simulink model "Robot"  (R2022b)
settings: Solver=FixedStepDiscrete  StartTime=0.0  StopTime=30  FixedStep=0.001  RelTol=1e-3
InitFcn:
  | load("BusConfig.mat");
undefined symbols (not defined in the file or in its folder): DiscIntNeverNeededParam
libraries: slrealtimeethercatlib x119, simulink x20
(part 6 of 7)

== system Robot/Motor3 Torque Control Init Frame/SDO Set 0x6098:35 Frame/If Action Subsystem6 ==
  In1 : Inport
  Action Port : ActionPort
  Out1 : Outport
  wires:
  In1/1 -> Out1/1

== system Robot/Motor3 Torque Control Init Frame/SDO Set 0x6098:35 Frame/If Action Subsystem7 ==
  In1 : Inport
  Action Port : ActionPort
  Discrete-Time Integrator : DiscreteIntegrator  SampleTime=-1  ICPrevOutput=DiscIntNeverNeededParam  ICPrevScaledInput=DiscIntNeverNeededParam
  Out1 : Outport
  wires:
  In1/1 -> Discrete-Time Integrator/1
  Discrete-Time Integrator/1 -> Out1/1

== system Robot/Motor3 Torque Control Init Frame/Set MasterState to OP Frame/If Action Subsystem5 ==
  In1 : Inport
  Action Port : ActionPort  ActionPortLabel=if((u1 > 0.1))
  Out1 : Outport
  wires:
  In1/1 -> Out1/1

== system Robot/Motor3 Torque Control Init Frame/Set MasterState to OP Frame/If Action Subsystem6 ==
  In1 : Inport
  Action Port : ActionPort  ActionPortLabel=else
  Out1 : Outport
  wires:
  In1/1 -> Out1/1

== system Robot/Motor3 Torque Control Init Frame/Set MasterState to OP Frame/If Action Subsystem7 ==
  In1 : Inport
  Action Port : ActionPort  ActionPortLabel=if((u1 == 8))
  Discrete-Time Integrator : DiscreteIntegrator  SampleTime=-1  ICPrevOutput=DiscIntNeverNeededParam  ICPrevScaledInput=DiscIntNeverNeededParam
  Out1 : Outport
  wires:
  In1/1 -> Discrete-Time Integrator/1
  Discrete-Time Integrator/1 -> Out1/1

== system Robot/Motor3 Torque Control Init Frame/Set MasterState to SafeOP Frame/If Action Subsystem5 ==
  In1 : Inport
  Action Port : ActionPort  ActionPortLabel=if((u1 > 0.1))
  Out1 : Outport
  wires:
  In1/1 -> Out1/1

== system Robot/Motor3 Torque Control Init Frame/Set MasterState to SafeOP Frame/If Action Subsystem6 ==
  In1 : Inport
  Action Port : ActionPort  ActionPortLabel=else
  Out1 : Outport
  wires:
  In1/1 -> Out1/1

== system Robot/Motor3 Torque Control Init Frame/Set MasterState to SafeOP Frame/If Action Subsystem7 ==
  In1 : Inport
  Action Port : ActionPort  ActionPortLabel=if((u1 == 4))
  Discrete-Time Integrator : DiscreteIntegrator  SampleTime=-1  ICPrevOutput=DiscIntNeverNeededParam  ICPrevScaledInput=DiscIntNeverNeededParam
  Out1 : Outport
  wires:
  In1/1 -> Discrete-Time Integrator/1
  Discrete-Time Integrator/1 -> Out1/1

== system Robot/Motor3 Torque Control Init Frame/State_10_Enable/Subsystem ==
  Case : Inport
  Case Default : Inport  Port=2
  Constant : Constant
  Constant1 : Constant  Value=0
  Constant2 : Constant  Value=TaskIndex
  Merge : Merge
  Switch Case Action Subsystem : Subsystem  TreatAsAtomicUnit=on
  Switch Case Action Subsystem1 : Subsystem  TreatAsAtomicUnit=on
  Enable : Outport
  FinishIndex : Outport  Port=2
  wires:
  Constant/1 -> Switch Case Action Subsystem/1(In1)
  Case/1 -> Switch Case Action Subsystem/Action
  Switch Case Action Subsystem/1(Out1) -> Merge/1
  Merge/1 -> Enable/1
  Case Default/1 -> Switch Case Action Subsystem1/Action
  Constant1/1 -> Switch Case Action Subsystem1/1(In1)
  Switch Case Action Subsystem1/1(Default) -> Merge/2
  Constant2/1 -> FinishIndex/1

== system Robot/Motor3 Torque Control Init Frame/State_11_Enable/Subsystem ==
  Case : Inport
  Case Default : Inport  Port=2
  Constant : Constant
  Constant1 : Constant  Value=0
  Constant2 : Constant  Value=TaskIndex
  Merge : Merge
  Switch Case Action Subsystem : Subsystem  TreatAsAtomicUnit=on
  Switch Case Action Subsystem1 : Subsystem  TreatAsAtomicUnit=on
  Enable : Outport
  FinishIndex : Outport  Port=2
  wires:
  Constant/1 -> Switch Case Action Subsystem/1(In1)
  Case/1 -> Switch Case Action Subsystem/Action
  Switch Case Action Subsystem/1(Out1) -> Merge/1
  Merge/1 -> Enable/1
  Case Default/1 -> Switch Case Action Subsystem1/Action
  Constant1/1 -> Switch Case Action Subsystem1/1(In1)
  Switch Case Action Subsystem1/1(Default) -> Merge/2
  Constant2/1 -> FinishIndex/1

== system Robot/Motor3 Torque Control Init Frame/State_12_Enable/Subsystem ==
  Case : Inport
  Case Default : Inport  Port=2
  Constant : Constant
  Constant1 : Constant  Value=0
  Constant2 : Constant  Value=TaskIndex
  Merge : Merge
  Switch Case Action Subsystem : Subsystem  TreatAsAtomicUnit=on
  Switch Case Action Subsystem1 : Subsystem  TreatAsAtomicUnit=on
  Enable : Outport
  FinishIndex : Outport  Port=2
  wires:
  Constant/1 -> Switch Case Action Subsystem/1(In1)
  Case/1 -> Switch Case Action Subsystem/Action
  Switch Case Action Subsystem/1(Out1) -> Merge/1
  Merge/1 -> Enable/1
  Case Default/1 -> Switch Case Action Subsystem1/Action
  Constant1/1 -> Switch Case Action Subsystem1/1(In1)
  Switch Case Action Subsystem1/1(Default) -> Merge/2
  Constant2/1 -> FinishIndex/1

== system Robot/Motor3 Torque Control Init Frame/State_13_Enable/Subsystem ==
  Case : Inport
  Case Default : Inport  Port=2
  Constant : Constant
  Constant1 : Constant  Value=0
  Constant2 : Constant  Value=TaskIndex
  Merge : Merge
  Switch Case Action Subsystem : Subsystem  TreatAsAtomicUnit=on
  Switch Case Action Subsystem1 : Subsystem  TreatAsAtomicUnit=on
  Enable : Outport
  FinishIndex : Outport  Port=2
  wires:
  Constant/1 -> Switch Case Action Subsystem/1(In1)
  Case/1 -> Switch Case Action Subsystem/Action
  Switch Case Action Subsystem/1(Out1) -> Merge/1
  Merge/1 -> Enable/1
  Case Default/1 -> Switch Case Action Subsystem1/Action
  Constant1/1 -> Switch Case Action Subsystem1/1(In1)
  Switch Case Action Subsystem1/1(Default) -> Merge/2
  Constant2/1 -> FinishIndex/1

== system Robot/Motor3 Torque Control Init Frame/State_1_Enable/Subsystem ==
  Case : Inport
  Case Default : Inport  Port=2
  Constant : Constant
  Constant1 : Constant  Value=0
  Constant2 : Constant  Value=TaskIndex
  Merge : Merge
  Switch Case Action Subsystem : Subsystem  TreatAsAtomicUnit=on
  Switch Case Action Subsystem1 : Subsystem  TreatAsAtomicUnit=on
  Enable : Outport
  FinishIndex : Outport  Port=2
  wires:
  Constant/1 -> Switch Case Action Subsystem/1(In1)
  Case/1 -> Switch Case Action Subsystem/Action
  Switch Case Action Subsystem/1(Out1) -> Merge/1
  Merge/1 -> Enable/1
  Case Default/1 -> Switch Case Action Subsystem1/Action
  Constant1/1 -> Switch Case Action Subsystem1/1(In1)
  Switch Case Action Subsystem1/1(Default) -> Merge/2
  Constant2/1 -> FinishIndex/1

== system Robot/Motor3 Torque Control Init Frame/State_2_Enable/Subsystem ==
  Case : Inport
  Case Default : Inport  Port=2
  Constant : Constant
  Constant1 : Constant  Value=0
  Constant2 : Constant  Value=TaskIndex
  Merge : Merge
  Switch Case Action Subsystem : Subsystem  TreatAsAtomicUnit=on
  Switch Case Action Subsystem1 : Subsystem  TreatAsAtomicUnit=on
  Enable : Outport
  FinishIndex : Outport  Port=2
  wires:
  Constant/1 -> Switch Case Action Subsystem/1(In1)
  Case/1 -> Switch Case Action Subsystem/Action
  Switch Case Action Subsystem/1(Out1) -> Merge/1
  Merge/1 -> Enable/1
  Case Default/1 -> Switch Case Action Subsystem1/Action
  Constant1/1 -> Switch Case Action Subsystem1/1(In1)
  Switch Case Action Subsystem1/1(Default) -> Merge/2
  Constant2/1 -> FinishIndex/1

== system Robot/Motor3 Torque Control Init Frame/State_3_Enable/Subsystem ==
  Case : Inport
  Case Default : Inport  Port=2
  Constant : Constant
  Constant1 : Constant  Value=0
  Constant2 : Constant  Value=TaskIndex
  Merge : Merge
  Switch Case Action Subsystem : Subsystem  TreatAsAtomicUnit=on
  Switch Case Action Subsystem1 : Subsystem  TreatAsAtomicUnit=on
  Enable : Outport
  FinishIndex : Outport  Port=2
  wires:
  Constant/1 -> Switch Case Action Subsystem/1(In1)
  Case/1 -> Switch Case Action Subsystem/Action
  Switch Case Action Subsystem/1(Out1) -> Merge/1
  Merge/1 -> Enable/1
  Case Default/1 -> Switch Case Action Subsystem1/Action
  Constant1/1 -> Switch Case Action Subsystem1/1(In1)
  Switch Case Action Subsystem1/1(Default) -> Merge/2
  Constant2/1 -> FinishIndex/1

== system Robot/Motor3 Torque Control Init Frame/State_4_Enable/Subsystem ==
  Case : Inport
  Case Default : Inport  Port=2
  Constant : Constant
  Constant1 : Constant  Value=0
  Constant2 : Constant  Value=TaskIndex
  Merge : Merge
  Switch Case Action Subsystem : Subsystem  TreatAsAtomicUnit=on
  Switch Case Action Subsystem1 : Subsystem  TreatAsAtomicUnit=on
  Enable : Outport
  FinishIndex : Outport  Port=2
  wires:
  Constant/1 -> Switch Case Action Subsystem/1(In1)
  Case/1 -> Switch Case Action Subsystem/Action
  Switch Case Action Subsystem/1(Out1) -> Merge/1
  Merge/1 -> Enable/1
  Case Default/1 -> Switch Case Action Subsystem1/Action
  Constant1/1 -> Switch Case Action Subsystem1/1(In1)
  Switch Case Action Subsystem1/1(Default) -> Merge/2
  Constant2/1 -> FinishIndex/1

== system Robot/Motor3 Torque Control Init Frame/State_5_Enable/Subsystem ==
  Case : Inport
  Case Default : Inport  Port=2
  Constant : Constant
  Constant1 : Constant  Value=0
  Constant2 : Constant  Value=TaskIndex
  Merge : Merge
  Switch Case Action Subsystem : Subsystem  TreatAsAtomicUnit=on
  Switch Case Action Subsystem1 : Subsystem  TreatAsAtomicUnit=on
  Enable : Outport
  FinishIndex : Outport  Port=2
  wires:
  Constant/1 -> Switch Case Action Subsystem/1(In1)
  Case/1 -> Switch Case Action Subsystem/Action
  Switch Case Action Subsystem/1(Out1) -> Merge/1
  Merge/1 -> Enable/1
  Case Default/1 -> Switch Case Action Subsystem1/Action
  Constant1/1 -> Switch Case Action Subsystem1/1(In1)
  Switch Case Action Subsystem1/1(Default) -> Merge/2
  Constant2/1 -> FinishIndex/1

== system Robot/Motor3 Torque Control Init Frame/State_6_Enable/Subsystem ==
  Case : Inport
  Case Default : Inport  Port=2
  Constant : Constant
  Constant1 : Constant  Value=0
  Constant2 : Constant  Value=TaskIndex
  Merge : Merge
  Switch Case Action Subsystem : Subsystem  TreatAsAtomicUnit=on
  Switch Case Action Subsystem1 : Subsystem  TreatAsAtomicUnit=on
  Enable : Outport
  FinishIndex : Outport  Port=2
  wires:
  Constant/1 -> Switch Case Action Subsystem/1(In1)
  Case/1 -> Switch Case Action Subsystem/Action
  Switch Case Action Subsystem/1(Out1) -> Merge/1
  Merge/1 -> Enable/1
  Case Default/1 -> Switch Case Action Subsystem1/Action
  Constant1/1 -> Switch Case Action Subsystem1/1(In1)
  Switch Case Action Subsystem1/1(Default) -> Merge/2
  Constant2/1 -> FinishIndex/1

== system Robot/Motor3 Torque Control Init Frame/State_7_Enable/Subsystem ==
  Case : Inport
  Case Default : Inport  Port=2
  Constant : Constant
  Constant1 : Constant  Value=0
  Constant2 : Constant  Value=TaskIndex
  Merge : Merge
  Switch Case Action Subsystem : Subsystem  TreatAsAtomicUnit=on
  Switch Case Action Subsystem1 : Subsystem  TreatAsAtomicUnit=on
  Enable : Outport
  FinishIndex : Outport  Port=2
  wires:
  Constant/1 -> Switch Case Action Subsystem/1(In1)
  Case/1 -> Switch Case Action Subsystem/Action
  Switch Case Action Subsystem/1(Out1) -> Merge/1
  Merge/1 -> Enable/1
  Case Default/1 -> Switch Case Action Subsystem1/Action
  Constant1/1 -> Switch Case Action Subsystem1/1(In1)
  Switch Case Action Subsystem1/1(Default) -> Merge/2
  Constant2/1 -> FinishIndex/1

== system Robot/Motor3 Torque Control Init Frame/State_8_Enable/Subsystem ==
  Case : Inport
  Case Default : Inport  Port=2
  Constant : Constant
  Constant1 : Constant  Value=0
  Constant2 : Constant  Value=TaskIndex
  Merge : Merge
  Switch Case Action Subsystem : Subsystem  TreatAsAtomicUnit=on
  Switch Case Action Subsystem1 : Subsystem  TreatAsAtomicUnit=on
  Enable : Outport
  FinishIndex : Outport  Port=2
  wires:
  Constant/1 -> Switch Case Action Subsystem/1(In1)
  Case/1 -> Switch Case Action Subsystem/Action
  Switch Case Action Subsystem/1(Out1) -> Merge/1
  Merge/1 -> Enable/1
  Case Default/1 -> Switch Case Action Subsystem1/Action
  Constant1/1 -> Switch Case Action Subsystem1/1(In1)
  Switch Case Action Subsystem1/1(Default) -> Merge/2
  Constant2/1 -> FinishIndex/1

== system Robot/Motor3 Torque Control Init Frame/State_9_Enable/Subsystem ==
  Case : Inport
  Case Default : Inport  Port=2
  Constant : Constant
  Constant1 : Constant  Value=0
  Constant2 : Constant  Value=TaskIndex
  Merge : Merge
  Switch Case Action Subsystem : Subsystem  TreatAsAtomicUnit=on
  Switch Case Action Subsystem1 : Subsystem  TreatAsAtomicUnit=on
  Enable : Outport
  FinishIndex : Outport  Port=2
  wires:
  Constant/1 -> Switch Case Action Subsystem/1(In1)
  Case/1 -> Switch Case Action Subsystem/Action
  Switch Case Action Subsystem/1(Out1) -> Merge/1
  Merge/1 -> Enable/1
  Case Default/1 -> Switch Case Action Subsystem1/Action
  Constant1/1 -> Switch Case Action Subsystem1/1(In1)
  Switch Case Action Subsystem1/1(Default) -> Merge/2
  Constant2/1 -> FinishIndex/1

== system Robot/Motor4 Torque Control Init Frame/Get MasterState OP Frame/If Action Subsystem5 ==
  In1 : Inport
  Action Port : ActionPort  ActionPortLabel=if((u1 == 8))
  Out1 : Outport
  wires:
  In1/1 -> Out1/1

== system Robot/Motor4 Torque Control Init Frame/Get MasterState OP Frame/If Action Subsystem6 ==
  In1 : Inport
  Action Port : ActionPort  ActionPortLabel=else
  Out1 : Outport
  wires:
  In1/1 -> Out1/1

== system Robot/Motor4 Torque Control Init Frame/Get MasterState OP Frame/If Action Subsystem7 ==
  In1 : Inport
  Action Port : ActionPort  ActionPortLabel=if((u1 == 4663))
  Discrete-Time Integrator : DiscreteIntegrator  SampleTime=-1  ICPrevOutput=DiscIntNeverNeededParam  ICPrevScaledInput=DiscIntNeverNeededParam
  Out1 : Outport
  wires:
  In1/1 -> Discrete-Time Integrator/1
  Discrete-Time Integrator/1 -> Out1/1

== system Robot/Motor4 Torque Control Init Frame/PDO Set 0x6040:6->7->15 Frame/If Action Subsystem ==
  In1 : Inport
  Action Port : ActionPort  ActionPortLabel=if((u1 == 720)&(u2 == 500))
  Out1 : Outport
  wires:
  In1/1 -> Out1/1

== system Robot/Motor4 Torque Control Init Frame/PDO Set 0x6040:6->7->15 Frame/If Action Subsystem1 ==
  In1 : Inport
  Action Port : ActionPort  ActionPortLabel=elseif((u1 == 689)&(u2 == 500))
  Out1 : Outport
  wires:
  In1/1 -> Out1/1

== system Robot/Motor4 Torque Control Init Frame/PDO Set 0x6040:6->7->15 Frame/If Action Subsystem2 ==
  In1 : Inport
  Action Port : ActionPort  ActionPortLabel=elseif( (u1 == 691)&(u2 == 500))
  Out1 : Outport
  wires:
  In1/1 -> Out1/1

== system Robot/Motor4 Torque Control Init Frame/PDO Set 0x6040:6->7->15 Frame/If Action Subsystem4 ==
  In1 : Inport
  Action Port : ActionPort  ActionPortLabel=else
  Out1 : Outport
  wires:
  In1/1 -> Out1/1

== system Robot/Motor4 Torque Control Init Frame/PDO Set 0x6040:6->7->15 Frame/If Action Subsystem5 ==
  In1 : Inport
  Action Port : ActionPort  ActionPortLabel=if((u1 >= 0.1))
  Out1 : Outport
  wires:
  In1/1 -> Out1/1

== system Robot/Motor4 Torque Control Init Frame/PDO Set 0x6040:6->7->15 Frame/If Action Subsystem6 ==
  In1 : Inport
  Action Port : ActionPort  ActionPortLabel=else
  Out1 : Outport
  wires:
  In1/1 -> Out1/1

== system Robot/Motor4 Torque Control Init Frame/PDO Set 0x6040:6->7->15 Frame/If Action Subsystem7 ==
  In1 : Inport
  Action Port : ActionPort  ActionPortLabel=if((u1 == 4663)|(u1 == 4791))
  Discrete-Time Integrator : DiscreteIntegrator  SampleTime=-1  ICPrevOutput=DiscIntNeverNeededParam  ICPrevScaledInput=DiscIntNeverNeededParam
  Out1 : Outport
  wires:
  In1/1 -> Discrete-Time Integrator/1
  Discrete-Time Integrator/1 -> Out1/1

== system Robot/Motor4 Torque Control Init Frame/SDO Get 0x6075 Frame/If Action Subsystem5 ==
  In1 : Inport
  Action Port : ActionPort  ActionPortLabel=if((u1 == 2))
  Out1 : Outport
  wires:
  In1/1 -> Out1/1

== system Robot/Motor4 Torque Control Init Frame/SDO Get 0x6075 Frame/If Action Subsystem6 ==
  In1 : Inport
  Action Port : ActionPort  ActionPortLabel=else
  Out1 : Outport
  wires:
  In1/1 -> Out1/1

== system Robot/Motor4 Torque Control Init Frame/SDO Get 0x6075 Frame/If Action Subsystem7 ==
  In1 : Inport
  Action Port : ActionPort  ActionPortLabel=if((u1 == 4663))
  Discrete-Time Integrator : DiscreteIntegrator  SampleTime=-1  ICPrevOutput=DiscIntNeverNeededParam  ICPrevScaledInput=DiscIntNeverNeededParam
  Out1 : Outport
  wires:
  In1/1 -> Discrete-Time Integrator/1
  Discrete-Time Integrator/1 -> Out1/1

== system Robot/Motor4 Torque Control Init Frame/SDO Set 0x6040:15 Frame/If Action Subsystem1 ==
  In1 : Inport
  Action Port : ActionPort
  Out1 : Outport
  wires:
  In1/1 -> Out1/1

== system Robot/Motor4 Torque Control Init Frame/SDO Set 0x6040:15 Frame/If Action Subsystem2 ==
  In1 : Inport
  Action Port : ActionPort
  Out1 : Outport
  wires:
  In1/1 -> Out1/1

== system Robot/Motor4 Torque Control Init Frame/SDO Set 0x6040:15 Frame/If Action Subsystem3 ==
  In1 : Inport
  Action Port : ActionPort
  Discrete-Time Integrator : DiscreteIntegrator  SampleTime=-1  ICPrevOutput=DiscIntNeverNeededParam  ICPrevScaledInput=DiscIntNeverNeededParam
  Out1 : Outport
  wires:
  In1/1 -> Discrete-Time Integrator/1
  Discrete-Time Integrator/1 -> Out1/1

== system Robot/Motor4 Torque Control Init Frame/SDO Set 0x6040:15 Frame/If Action Subsystem5 ==
  In1 : Inport
  Action Port : ActionPort
  Out1 : Outport
  wires:
  In1/1 -> Out1/1

== system Robot/Motor4 Torque Control Init Frame/SDO Set 0x6040:15 Frame/If Action Subsystem6 ==
  In1 : Inport
  Action Port : ActionPort
  Out1 : Outport
  wires:
  In1/1 -> Out1/1

== system Robot/Motor4 Torque Control Init Frame/SDO Set 0x6040:15 Frame/If Action Subsystem7 ==
  In1 : Inport
  Action Port : ActionPort
  Discrete-Time Integrator : DiscreteIntegrator  SampleTime=-1  ICPrevOutput=DiscIntNeverNeededParam  ICPrevScaledInput=DiscIntNeverNeededParam
  Out1 : Outport
  wires:
  In1/1 -> Discrete-Time Integrator/1
  Discrete-Time Integrator/1 -> Out1/1

== system Robot/Motor4 Torque Control Init Frame/SDO Set 0x6040:31 Frame/If Action Subsystem1 ==
  In1 : Inport
  Action Port : ActionPort
  Out1 : Outport
  wires:
  In1/1 -> Out1/1

== system Robot/Motor4 Torque Control Init Frame/SDO Set 0x6040:31 Frame/If Action Subsystem2 ==
  In1 : Inport
  Action Port : ActionPort
  Out1 : Outport
  wires:
  In1/1 -> Out1/1

== system Robot/Motor4 Torque Control Init Frame/SDO Set 0x6040:31 Frame/If Action Subsystem3 ==
  In1 : Inport
  Action Port : ActionPort
  Discrete-Time Integrator : DiscreteIntegrator  SampleTime=-1  ICPrevOutput=DiscIntNeverNeededParam  ICPrevScaledInput=DiscIntNeverNeededParam
  Out1 : Outport
  wires:
  In1/1 -> Discrete-Time Integrator/1
  Discrete-Time Integrator/1 -> Out1/1

== system Robot/Motor4 Torque Control Init Frame/SDO Set 0x6040:31 Frame/If Action Subsystem5 ==
  In1 : Inport
  Action Port : ActionPort
  Out1 : Outport
  wires:
  In1/1 -> Out1/1

== system Robot/Motor4 Torque Control Init Frame/SDO Set 0x6040:31 Frame/If Action Subsystem6 ==
  In1 : Inport
  Action Port : ActionPort
  Out1 : Outport
  wires:
  In1/1 -> Out1/1

== system Robot/Motor4 Torque Control Init Frame/SDO Set 0x6040:31 Frame/If Action Subsystem7 ==
  In1 : Inport
  Action Port : ActionPort
  Discrete-Time Integrator : DiscreteIntegrator  SampleTime=-1  ICPrevOutput=DiscIntNeverNeededParam  ICPrevScaledInput=DiscIntNeverNeededParam
  Out1 : Outport
  wires:
  In1/1 -> Discrete-Time Integrator/1
  Discrete-Time Integrator/1 -> Out1/1

== system Robot/Motor4 Torque Control Init Frame/SDO Set 0x6040:6 Frame/If Action Subsystem1 ==
  In1 : Inport
  Action Port : ActionPort
  Out1 : Outport
  wires:
  In1/1 -> Out1/1

== system Robot/Motor4 Torque Control Init Frame/SDO Set 0x6040:6 Frame/If Action Subsystem2 ==
  In1 : Inport
  Action Port : ActionPort
  Out1 : Outport
  wires:
  In1/1 -> Out1/1

== system Robot/Motor4 Torque Control Init Frame/SDO Set 0x6040:6 Frame/If Action Subsystem3 ==
  In1 : Inport
  Action Port : ActionPort
  Discrete-Time Integrator : DiscreteIntegrator  SampleTime=-1  ICPrevOutput=DiscIntNeverNeededParam  ICPrevScaledInput=DiscIntNeverNeededParam
  Out1 : Outport
  wires:
  In1/1 -> Discrete-Time Integrator/1
  Discrete-Time Integrator/1 -> Out1/1

== system Robot/Motor4 Torque Control Init Frame/SDO Set 0x6040:6 Frame/If Action Subsystem5 ==
  In1 : Inport
  Action Port : ActionPort
  Out1 : Outport
  wires:
  In1/1 -> Out1/1

== system Robot/Motor4 Torque Control Init Frame/SDO Set 0x6040:6 Frame/If Action Subsystem6 ==
  In1 : Inport
  Action Port : ActionPort
  Out1 : Outport
  wires:
  In1/1 -> Out1/1

== system Robot/Motor4 Torque Control Init Frame/SDO Set 0x6040:6 Frame/If Action Subsystem7 ==
  In1 : Inport
  Action Port : ActionPort
  Discrete-Time Integrator : DiscreteIntegrator  SampleTime=-1  ICPrevOutput=DiscIntNeverNeededParam  ICPrevScaledInput=DiscIntNeverNeededParam
  Out1 : Outport
  wires:
  In1/1 -> Discrete-Time Integrator/1
  Discrete-Time Integrator/1 -> Out1/1

== system Robot/Motor4 Torque Control Init Frame/SDO Set 0x6040:7 Frame/If Action Subsystem1 ==
  In1 : Inport
  Action Port : ActionPort
  Out1 : Outport
  wires:
  In1/1 -> Out1/1

== system Robot/Motor4 Torque Control Init Frame/SDO Set 0x6040:7 Frame/If Action Subsystem2 ==
  In1 : Inport
  Action Port : ActionPort
  Out1 : Outport
  wires:
  In1/1 -> Out1/1

== system Robot/Motor4 Torque Control Init Frame/SDO Set 0x6040:7 Frame/If Action Subsystem3 ==
  In1 : Inport
  Action Port : ActionPort
  Discrete-Time Integrator : DiscreteIntegrator  SampleTime=-1  ICPrevOutput=DiscIntNeverNeededParam  ICPrevScaledInput=DiscIntNeverNeededParam
  Out1 : Outport
  wires:
  In1/1 -> Discrete-Time Integrator/1
  Discrete-Time Integrator/1 -> Out1/1

== system Robot/Motor4 Torque Control Init Frame/SDO Set 0x6040:7 Frame/If Action Subsystem5 ==
  In1 : Inport
  Action Port : ActionPort
  Out1 : Outport
  wires:
  In1/1 -> Out1/1

== system Robot/Motor4 Torque Control Init Frame/SDO Set 0x6040:7 Frame/If Action Subsystem6 ==
  In1 : Inport
  Action Port : ActionPort
  Out1 : Outport
  wires:
  In1/1 -> Out1/1

== system Robot/Motor4 Torque Control Init Frame/SDO Set 0x6040:7 Frame/If Action Subsystem7 ==
  In1 : Inport
  Action Port : ActionPort
  Discrete-Time Integrator : DiscreteIntegrator  SampleTime=-1  ICPrevOutput=DiscIntNeverNeededParam  ICPrevScaledInput=DiscIntNeverNeededParam
  Out1 : Outport
  wires:
  In1/1 -> Discrete-Time Integrator/1
  Discrete-Time Integrator/1 -> Out1/1

== system Robot/Motor4 Torque Control Init Frame/SDO Set 0x6060:10 Frame/If Action Subsystem5 ==
  In1 : Inport
  Action Port : ActionPort  ActionPortLabel=if((u1 == 2))
  Out1 : Outport
  wires:
  In1/1 -> Out1/1

== system Robot/Motor4 Torque Control Init Frame/SDO Set 0x6060:10 Frame/If Action Subsystem6 ==
  In1 : Inport
  Action Port : ActionPort  ActionPortLabel=else
  Out1 : Outport
  wires:
  In1/1 -> Out1/1

== system Robot/Motor4 Torque Control Init Frame/SDO Set 0x6060:10 Frame/If Action Subsystem7 ==
  In1 : Inport
  Action Port : ActionPort  ActionPortLabel=if((u1 == 4663))
  Discrete-Time Integrator : DiscreteIntegrator  SampleTime=-1  ICPrevOutput=DiscIntNeverNeededParam  ICPrevScaledInput=DiscIntNeverNeededParam
  Out1 : Outport
  wires:
  In1/1 -> Discrete-Time Integrator/1
  Discrete-Time Integrator/1 -> Out1/1

== system Robot/Motor4 Torque Control Init Frame/SDO Set 0x6060:6 Frame/If Action Subsystem5 ==
  In1 : Inport
  Action Port : ActionPort
  Out1 : Outport
  wires:
  In1/1 -> Out1/1

== system Robot/Motor4 Torque Control Init Frame/SDO Set 0x6060:6 Frame/If Action Subsystem6 ==
  In1 : Inport
  Action Port : ActionPort
  Out1 : Outport
  wires:
  In1/1 -> Out1/1

== system Robot/Motor4 Torque Control Init Frame/SDO Set 0x6060:6 Frame/If Action Subsystem7 ==
  In1 : Inport
  Action Port : ActionPort
  Discrete-Time Integrator : DiscreteIntegrator  SampleTime=-1  ICPrevOutput=DiscIntNeverNeededParam  ICPrevScaledInput=DiscIntNeverNeededParam
  Out1 : Outport
  wires:
  In1/1 -> Discrete-Time Integrator/1
  Discrete-Time Integrator/1 -> Out1/1

== system Robot/Motor4 Torque Control Init Frame/SDO Set 0x6080:-1 Frame/If Action Subsystem5 ==
  In1 : Inport
  Action Port : ActionPort  ActionPortLabel=if((u1 == 2))
  Out1 : Outport
  wires:
  In1/1 -> Out1/1

== system Robot/Motor4 Torque Control Init Frame/SDO Set 0x6080:-1 Frame/If Action Subsystem6 ==
  In1 : Inport
  Action Port : ActionPort  ActionPortLabel=else
  Out1 : Outport
  wires:
  In1/1 -> Out1/1

== system Robot/Motor4 Torque Control Init Frame/SDO Set 0x6080:-1 Frame/If Action Subsystem7 ==
  In1 : Inport
  Action Port : ActionPort  ActionPortLabel=if((u1 == 4663))
  Discrete-Time Integrator : DiscreteIntegrator  SampleTime=-1  ICPrevOutput=DiscIntNeverNeededParam  ICPrevScaledInput=DiscIntNeverNeededParam
  Out1 : Outport
  wires:
  In1/1 -> Discrete-Time Integrator/1
  Discrete-Time Integrator/1 -> Out1/1

== system Robot/Motor4 Torque Control Init Frame/SDO Set 0x6098:35 Frame/If Action Subsystem5 ==
  In1 : Inport
  Action Port : ActionPort
  Out1 : Outport
  wires:
  In1/1 -> Out1/1

== system Robot/Motor4 Torque Control Init Frame/SDO Set 0x6098:35 Frame/If Action Subsystem6 ==
  In1 : Inport
  Action Port : ActionPort
  Out1 : Outport
  wires:
  In1/1 -> Out1/1

== system Robot/Motor4 Torque Control Init Frame/SDO Set 0x6098:35 Frame/If Action Subsystem7 ==
  In1 : Inport
  Action Port : ActionPort
  Discrete-Time Integrator : DiscreteIntegrator  SampleTime=-1  ICPrevOutput=DiscIntNeverNeededParam  ICPrevScaledInput=DiscIntNeverNeededParam
  Out1 : Outport
  wires:
  In1/1 -> Discrete-Time Integrator/1
  Discrete-Time Integrator/1 -> Out1/1

== system Robot/Motor4 Torque Control Init Frame/Set MasterState to OP Frame/If Action Subsystem5 ==
  In1 : Inport
  Action Port : ActionPort  ActionPortLabel=if((u1 > 0.1))
  Out1 : Outport
  wires:
  In1/1 -> Out1/1

== system Robot/Motor4 Torque Control Init Frame/Set MasterState to OP Frame/If Action Subsystem6 ==
  In1 : Inport
  Action Port : ActionPort  ActionPortLabel=else
  Out1 : Outport
  wires:
  In1/1 -> Out1/1

== system Robot/Motor4 Torque Control Init Frame/Set MasterState to OP Frame/If Action Subsystem7 ==
  In1 : Inport
  Action Port : ActionPort  ActionPortLabel=if((u1 == 8))
  Discrete-Time Integrator : DiscreteIntegrator  SampleTime=-1  ICPrevOutput=DiscIntNeverNeededParam  ICPrevScaledInput=DiscIntNeverNeededParam
  Out1 : Outport
  wires:
  In1/1 -> Discrete-Time Integrator/1
  Discrete-Time Integrator/1 -> Out1/1

== system Robot/Motor4 Torque Control Init Frame/Set MasterState to SafeOP Frame/If Action Subsystem5 ==
  In1 : Inport
  Action Port : ActionPort  ActionPortLabel=if((u1 > 0.1))
  Out1 : Outport
  wires:
  In1/1 -> Out1/1

== system Robot/Motor4 Torque Control Init Frame/Set MasterState to SafeOP Frame/If Action Subsystem6 ==
  In1 : Inport
  Action Port : ActionPort  ActionPortLabel=else
  Out1 : Outport
  wires:
  In1/1 -> Out1/1

== system Robot/Motor4 Torque Control Init Frame/Set MasterState to SafeOP Frame/If Action Subsystem7 ==
  In1 : Inport
  Action Port : ActionPort  ActionPortLabel=if((u1 == 4))
  Discrete-Time Integrator : DiscreteIntegrator  SampleTime=-1  ICPrevOutput=DiscIntNeverNeededParam  ICPrevScaledInput=DiscIntNeverNeededParam
  Out1 : Outport
  wires:
  In1/1 -> Discrete-Time Integrator/1
  Discrete-Time Integrator/1 -> Out1/1

== system Robot/Motor4 Torque Control Init Frame/State_10_Enable/Subsystem ==
  Case : Inport
  Case Default : Inport  Port=2
  Constant : Constant
  Constant1 : Constant  Value=0
  Constant2 : Constant  Value=TaskIndex
  Merge : Merge
  Switch Case Action Subsystem : Subsystem  TreatAsAtomicUnit=on
  Switch Case Action Subsystem1 : Subsystem  TreatAsAtomicUnit=on
  Enable : Outport
  FinishIndex : Outport  Port=2
  wires:
  Constant/1 -> Switch Case Action Subsystem/1(In1)
  Case/1 -> Switch Case Action Subsystem/Action
  Switch Case Action Subsystem/1(Out1) -> Merge/1
  Merge/1 -> Enable/1
  Case Default/1 -> Switch Case Action Subsystem1/Action
  Constant1/1 -> Switch Case Action Subsystem1/1(In1)
  Switch Case Action Subsystem1/1(Default) -> Merge/2
  Constant2/1 -> FinishIndex/1

== system Robot/Motor4 Torque Control Init Frame/State_11_Enable/Subsystem ==
  Case : Inport
  Case Default : Inport  Port=2
  Constant : Constant
  Constant1 : Constant  Value=0
  Constant2 : Constant  Value=TaskIndex
  Merge : Merge
  Switch Case Action Subsystem : Subsystem  TreatAsAtomicUnit=on
  Switch Case Action Subsystem1 : Subsystem  TreatAsAtomicUnit=on
  Enable : Outport
  FinishIndex : Outport  Port=2
  wires:
  Constant/1 -> Switch Case Action Subsystem/1(In1)
  Case/1 -> Switch Case Action Subsystem/Action
  Switch Case Action Subsystem/1(Out1) -> Merge/1
  Merge/1 -> Enable/1
  Case Default/1 -> Switch Case Action Subsystem1/Action
  Constant1/1 -> Switch Case Action Subsystem1/1(In1)
  Switch Case Action Subsystem1/1(Default) -> Merge/2
  Constant2/1 -> FinishIndex/1

== system Robot/Motor4 Torque Control Init Frame/State_12_Enable/Subsystem ==
  Case : Inport
  Case Default : Inport  Port=2
  Constant : Constant
  Constant1 : Constant  Value=0
  Constant2 : Constant  Value=TaskIndex
  Merge : Merge
  Switch Case Action Subsystem : Subsystem  TreatAsAtomicUnit=on
  Switch Case Action Subsystem1 : Subsystem  TreatAsAtomicUnit=on
  Enable : Outport
  FinishIndex : Outport  Port=2
  wires:
  Constant/1 -> Switch Case Action Subsystem/1(In1)
  Case/1 -> Switch Case Action Subsystem/Action
  Switch Case Action Subsystem/1(Out1) -> Merge/1
  Merge/1 -> Enable/1
  Case Default/1 -> Switch Case Action Subsystem1/Action
  Constant1/1 -> Switch Case Action Subsystem1/1(In1)
  Switch Case Action Subsystem1/1(Default) -> Merge/2
  Constant2/1 -> FinishIndex/1

== system Robot/Motor4 Torque Control Init Frame/State_13_Enable/Subsystem ==
  Case : Inport
  Case Default : Inport  Port=2
  Constant : Constant
  Constant1 : Constant  Value=0
  Constant2 : Constant  Value=TaskIndex
  Merge : Merge
  Switch Case Action Subsystem : Subsystem  TreatAsAtomicUnit=on
  Switch Case Action Subsystem1 : Subsystem  TreatAsAtomicUnit=on
  Enable : Outport
  FinishIndex : Outport  Port=2
  wires:
  Constant/1 -> Switch Case Action Subsystem/1(In1)
  Case/1 -> Switch Case Action Subsystem/Action
  Switch Case Action Subsystem/1(Out1) -> Merge/1
  Merge/1 -> Enable/1
  Case Default/1 -> Switch Case Action Subsystem1/Action
  Constant1/1 -> Switch Case Action Subsystem1/1(In1)
  Switch Case Action Subsystem1/1(Default) -> Merge/2
  Constant2/1 -> FinishIndex/1

== system Robot/Motor4 Torque Control Init Frame/State_1_Enable/Subsystem ==
  Case : Inport
  Case Default : Inport  Port=2
  Constant : Constant
  Constant1 : Constant  Value=0
  Constant2 : Constant  Value=TaskIndex
  Merge : Merge
  Switch Case Action Subsystem : Subsystem  TreatAsAtomicUnit=on
  Switch Case Action Subsystem1 : Subsystem  TreatAsAtomicUnit=on
  Enable : Outport
  FinishIndex : Outport  Port=2
  wires:
  Constant/1 -> Switch Case Action Subsystem/1(In1)
  Case/1 -> Switch Case Action Subsystem/Action
  Switch Case Action Subsystem/1(Out1) -> Merge/1
  Merge/1 -> Enable/1
  Case Default/1 -> Switch Case Action Subsystem1/Action
  Constant1/1 -> Switch Case Action Subsystem1/1(In1)
  Switch Case Action Subsystem1/1(Default) -> Merge/2
  Constant2/1 -> FinishIndex/1

== system Robot/Motor4 Torque Control Init Frame/State_2_Enable/Subsystem ==
  Case : Inport
  Case Default : Inport  Port=2
  Constant : Constant
  Constant1 : Constant  Value=0
  Constant2 : Constant  Value=TaskIndex
  Merge : Merge
  Switch Case Action Subsystem : Subsystem  TreatAsAtomicUnit=on
  Switch Case Action Subsystem1 : Subsystem  TreatAsAtomicUnit=on
  Enable : Outport
  FinishIndex : Outport  Port=2
  wires:
  Constant/1 -> Switch Case Action Subsystem/1(In1)
  Case/1 -> Switch Case Action Subsystem/Action
  Switch Case Action Subsystem/1(Out1) -> Merge/1
  Merge/1 -> Enable/1
  Case Default/1 -> Switch Case Action Subsystem1/Action
  Constant1/1 -> Switch Case Action Subsystem1/1(In1)
  Switch Case Action Subsystem1/1(Default) -> Merge/2
  Constant2/1 -> FinishIndex/1

== system Robot/Motor4 Torque Control Init Frame/State_3_Enable/Subsystem ==
  Case : Inport
  Case Default : Inport  Port=2
  Constant : Constant
  Constant1 : Constant  Value=0
  Constant2 : Constant  Value=TaskIndex
  Merge : Merge
  Switch Case Action Subsystem : Subsystem  TreatAsAtomicUnit=on
  Switch Case Action Subsystem1 : Subsystem  TreatAsAtomicUnit=on
  Enable : Outport
  FinishIndex : Outport  Port=2
  wires:
  Constant/1 -> Switch Case Action Subsystem/1(In1)
  Case/1 -> Switch Case Action Subsystem/Action
  Switch Case Action Subsystem/1(Out1) -> Merge/1
  Merge/1 -> Enable/1
  Case Default/1 -> Switch Case Action Subsystem1/Action
  Constant1/1 -> Switch Case Action Subsystem1/1(In1)
  Switch Case Action Subsystem1/1(Default) -> Merge/2
  Constant2/1 -> FinishIndex/1

== system Robot/Motor4 Torque Control Init Frame/State_4_Enable/Subsystem ==
  Case : Inport
  Case Default : Inport  Port=2
  Constant : Constant
  Constant1 : Constant  Value=0
  Constant2 : Constant  Value=TaskIndex
  Merge : Merge
  Switch Case Action Subsystem : Subsystem  TreatAsAtomicUnit=on
  Switch Case Action Subsystem1 : Subsystem  TreatAsAtomicUnit=on
  Enable : Outport
  FinishIndex : Outport  Port=2
  wires:
  Constant/1 -> Switch Case Action Subsystem/1(In1)
  Case/1 -> Switch Case Action Subsystem/Action
  Switch Case Action Subsystem/1(Out1) -> Merge/1
  Merge/1 -> Enable/1
  Case Default/1 -> Switch Case Action Subsystem1/Action
  Constant1/1 -> Switch Case Action Subsystem1/1(In1)
  Switch Case Action Subsystem1/1(Default) -> Merge/2
  Constant2/1 -> FinishIndex/1

== system Robot/Motor4 Torque Control Init Frame/State_5_Enable/Subsystem ==
  Case : Inport
  Case Default : Inport  Port=2
  Constant : Constant
  Constant1 : Constant  Value=0
  Constant2 : Constant  Value=TaskIndex
  Merge : Merge
  Switch Case Action Subsystem : Subsystem  TreatAsAtomicUnit=on
  Switch Case Action Subsystem1 : Subsystem  TreatAsAtomicUnit=on
  Enable : Outport
  FinishIndex : Outport  Port=2
  wires:
  Constant/1 -> Switch Case Action Subsystem/1(In1)
  Case/1 -> Switch Case Action Subsystem/Action
  Switch Case Action Subsystem/1(Out1) -> Merge/1
  Merge/1 -> Enable/1
  Case Default/1 -> Switch Case Action Subsystem1/Action
  Constant1/1 -> Switch Case Action Subsystem1/1(In1)
  Switch Case Action Subsystem1/1(Default) -> Merge/2
  Constant2/1 -> FinishIndex/1

== system Robot/Motor4 Torque Control Init Frame/State_6_Enable/Subsystem ==
  Case : Inport
  Case Default : Inport  Port=2
  Constant : Constant
  Constant1 : Constant  Value=0
  Constant2 : Constant  Value=TaskIndex
  Merge : Merge
  Switch Case Action Subsystem : Subsystem  TreatAsAtomicUnit=on
  Switch Case Action Subsystem1 : Subsystem  TreatAsAtomicUnit=on
  Enable : Outport
  FinishIndex : Outport  Port=2
  wires:
  Constant/1 -> Switch Case Action Subsystem/1(In1)
  Case/1 -> Switch Case Action Subsystem/Action
  Switch Case Action Subsystem/1(Out1) -> Merge/1
  Merge/1 -> Enable/1
  Case Default/1 -> Switch Case Action Subsystem1/Action
  Constant1/1 -> Switch Case Action Subsystem1/1(In1)
  Switch Case Action Subsystem1/1(Default) -> Merge/2
  Constant2/1 -> FinishIndex/1

== system Robot/Motor4 Torque Control Init Frame/State_7_Enable/Subsystem ==
  Case : Inport
  Case Default : Inport  Port=2
  Constant : Constant
  Constant1 : Constant  Value=0
  Constant2 : Constant  Value=TaskIndex
  Merge : Merge
  Switch Case Action Subsystem : Subsystem  TreatAsAtomicUnit=on
  Switch Case Action Subsystem1 : Subsystem  TreatAsAtomicUnit=on
  Enable : Outport
  FinishIndex : Outport  Port=2
  wires:
  Constant/1 -> Switch Case Action Subsystem/1(In1)
  Case/1 -> Switch Case Action Subsystem/Action
  Switch Case Action Subsystem/1(Out1) -> Merge/1
  Merge/1 -> Enable/1
  Case Default/1 -> Switch Case Action Subsystem1/Action
  Constant1/1 -> Switch Case Action Subsystem1/1(In1)
  Switch Case Action Subsystem1/1(Default) -> Merge/2
  Constant2/1 -> FinishIndex/1

== system Robot/Motor4 Torque Control Init Frame/State_8_Enable/Subsystem ==
  Case : Inport
  Case Default : Inport  Port=2
  Constant : Constant
  Constant1 : Constant  Value=0
  Constant2 : Constant  Value=TaskIndex
  Merge : Merge
  Switch Case Action Subsystem : Subsystem  TreatAsAtomicUnit=on
  Switch Case Action Subsystem1 : Subsystem  TreatAsAtomicUnit=on
  Enable : Outport
  FinishIndex : Outport  Port=2
  wires:
  Constant/1 -> Switch Case Action Subsystem/1(In1)
  Case/1 -> Switch Case Action Subsystem/Action
  Switch Case Action Subsystem/1(Out1) -> Merge/1
  Merge/1 -> Enable/1
  Case Default/1 -> Switch Case Action Subsystem1/Action
  Constant1/1 -> Switch Case Action Subsystem1/1(In1)
  Switch Case Action Subsystem1/1(Default) -> Merge/2
  Constant2/1 -> FinishIndex/1

== system Robot/Motor4 Torque Control Init Frame/State_9_Enable/Subsystem ==
  Case : Inport
  Case Default : Inport  Port=2
  Constant : Constant
  Constant1 : Constant  Value=0
  Constant2 : Constant  Value=TaskIndex
  Merge : Merge
  Switch Case Action Subsystem : Subsystem  TreatAsAtomicUnit=on
  Switch Case Action Subsystem1 : Subsystem  TreatAsAtomicUnit=on
  Enable : Outport
  FinishIndex : Outport  Port=2
  wires:
  Constant/1 -> Switch Case Action Subsystem/1(In1)
  Case/1 -> Switch Case Action Subsystem/Action
  Switch Case Action Subsystem/1(Out1) -> Merge/1
  Merge/1 -> Enable/1
  Case Default/1 -> Switch Case Action Subsystem1/Action
  Constant1/1 -> Switch Case Action Subsystem1/1(In1)
  Switch Case Action Subsystem1/1(Default) -> Merge/2
  Constant2/1 -> FinishIndex/1

== system Robot/State_1_Enable/Subsystem/Switch Case Action Subsystem ==
  In1 : Inport
  Action Port : ActionPort  ActionPortLabel=case [ 1 ]:
  Out1 : Outport
  wires:
  In1/1 -> Out1/1

== system Robot/State_1_Enable/Subsystem/Switch Case Action Subsystem1 ==
  In1 : Inport
  Action Port : ActionPort  ActionPortLabel=default:
  Default : Outport
  wires:
  In1/1 -> Default/1

== system Robot/State_2_Enable/Subsystem/Switch Case Action Subsystem ==
  In1 : Inport
  Action Port : ActionPort  ActionPortLabel=case [ 2 ]:
  Out1 : Outport
  wires:
  In1/1 -> Out1/1

== system Robot/State_2_Enable/Subsystem/Switch Case Action Subsystem1 ==
  In1 : Inport
  Action Port : ActionPort  ActionPortLabel=default:
  Default : Outport
  wires:
  In1/1 -> Default/1

== system Robot/State_3_Enable/Subsystem/Switch Case Action Subsystem ==
  In1 : Inport
  Action Port : ActionPort  ActionPortLabel=case [ 3 ]:
  Out1 : Outport
  wires:
  In1/1 -> Out1/1

== system Robot/State_3_Enable/Subsystem/Switch Case Action Subsystem1 ==
  In1 : Inport
  Action Port : ActionPort  ActionPortLabel=default:
  Default : Outport
  wires:
  In1/1 -> Default/1

== system Robot/State_4_Enable/Subsystem/Switch Case Action Subsystem ==
  In1 : Inport
  Action Port : ActionPort  ActionPortLabel=case [ 4 ]:
  Out1 : Outport
  wires:
  In1/1 -> Out1/1

== system Robot/State_4_Enable/Subsystem/Switch Case Action Subsystem1 ==
  In1 : Inport
  Action Port : ActionPort  ActionPortLabel=default:
  Default : Outport
  wires:
  In1/1 -> Default/1

== system Robot/State_5_Enable/Subsystem/Switch Case Action Subsystem ==
  In1 : Inport
  Action Port : ActionPort  ActionPortLabel=case [ 5 ]:
  Out1 : Outport
  wires:
  In1/1 -> Out1/1

== system Robot/State_5_Enable/Subsystem/Switch Case Action Subsystem1 ==
  In1 : Inport
  Action Port : ActionPort  ActionPortLabel=default:
  Default : Outport
  wires:
  In1/1 -> Default/1

== system Robot/Subsystem/Robot/Motor1 ==
  DesireTorque : Inport
  EtherCAT PDO Receive1 : slrealtimeethercatlib/EtherCAT PDO Receive  Priority=2  sig_name=Drive 1 (Elmo Drive ).Inputs.Position actual value  sig_offset=696  sig_type=int32  type_size=32  sig_dim=1  device_id=0  sample_time=0.001000
  EtherCAT PDO Receive2 : slrealtimeethercatlib/EtherCAT PDO Receive  Priority=2  sig_name=Drive 1 (Elmo Drive ).Inputs_1.Velocity actual value  sig_offset=776  sig_type=int32  type_size=32  sig_dim=1  device_id=0  sample_time=0.001000
  EtherCAT PDO Receive3 : slrealtimeethercatlib/EtherCAT PDO Receive  Priority=2  sig_name=Drive 1 (Elmo Drive ).Inputs.Torque actual value  sig_offset=728  sig_type=int16  type_size=16  sig_dim=1  device_id=0  sample_time=0.001000
  EtherCAT PDO Receive4 : slrealtimeethercatlib/EtherCAT PDO Receive  Priority=2  sig_name=Drive 1 (Elmo Drive ).Inputs_2.DC link circuit voltage  sig_offset=808  sig_type=uint32  type_size=32  sig_dim=1  device_id=0  sample_time=0.001000
  EtherCAT PDO Receive5 : slrealtimeethercatlib/EtherCAT PDO Receive  Priority=2  sig_name=Drive 1 (Elmo Drive ).Inputs.Mode of operation display  sig_offset=760  sig_type=int8  type_size=8  sig_dim=1  device_id=0  sample_time=0.001000
  EtherCAT PDO Transmit : slrealtimeethercatlib/EtherCAT PDO Transmit  Priority=5  sig_name=Drive 1 (Elmo Drive ).Outputs.Target Torque  sig_offset=696  sig_type=int16  type_size=16  sig_dim=1  device_id=0  sample_time=0.001000
  ActuralPosition : Outport
  ActuralVelocity : Outport  Port=2
  ActuralTorque : Outport  Port=3
  DCLinkCircuitVoltage : Outport  Port=4
  ModeofOperationDisplay : Outport  Port=5
  wires:
  EtherCAT PDO Receive4/1 -> DCLinkCircuitVoltage/1
  EtherCAT PDO Receive3/1 -> ActuralTorque/1
  EtherCAT PDO Receive5/1 -> ModeofOperationDisplay/1
  DesireTorque/1 -> EtherCAT PDO Transmit/1
  EtherCAT PDO Receive1/1 -> ActuralPosition/1
  EtherCAT PDO Receive2/1 -> ActuralVelocity/1

== system Robot/Subsystem/Robot/Motor2 ==
  DesireTorque : Inport
  EtherCAT PDO Receive1 : slrealtimeethercatlib/EtherCAT PDO Receive  Priority=2  sig_name=Drive 2 (Elmo Drive ).Inputs.Position actual value  sig_offset=12496  sig_type=int32  type_size=32  sig_dim=1  device_id=0  sample_time=0.001000
  EtherCAT PDO Receive2 : slrealtimeethercatlib/EtherCAT PDO Receive  Priority=2  sig_name=Drive 2 (Elmo Drive ).Inputs_1.Velocity actual value  sig_offset=12576  sig_type=int32  type_size=32  sig_dim=1  device_id=0  sample_time=0.001000
  EtherCAT PDO Receive3 : slrealtimeethercatlib/EtherCAT PDO Receive  Priority=2  sig_name=Drive 2 (Elmo Drive ).Inputs.Torque actual value  sig_offset=12528  sig_type=int16  type_size=16  sig_dim=1  device_id=0  sample_time=0.001000
  EtherCAT PDO Receive4 : slrealtimeethercatlib/EtherCAT PDO Receive  Priority=2  sig_name=Drive 2 (Elmo Drive ).Inputs_2.DC link circuit voltage  sig_offset=12608  sig_type=uint32  type_size=32  sig_dim=1  device_id=0  sample_time=0.001000
  EtherCAT PDO Receive5 : slrealtimeethercatlib/EtherCAT PDO Receive  Priority=2  sig_name=Drive 2 (Elmo Drive ).Inputs.Mode of operation display  sig_offset=12560  sig_type=int8  type_size=8  sig_dim=1  device_id=0  sample_time=0.001000
  EtherCAT PDO Transmit : slrealtimeethercatlib/EtherCAT PDO Transmit  Priority=5  sig_name=Drive 2 (Elmo Drive ).Outputs.Target Torque  sig_offset=12496  sig_type=int16  type_size=16  sig_dim=1  device_id=0  sample_time=0.001000
  ActuralPosition : Outport
  ActuralVelocity : Outport  Port=2
  ActuralTorque : Outport  Port=3
  DCLinkCircuitVoltage : Outport  Port=4
  ModeofOperationDisplay : Outport  Port=5
  wires:
  EtherCAT PDO Receive4/1 -> DCLinkCircuitVoltage/1
  EtherCAT PDO Receive3/1 -> ActuralTorque/1
  EtherCAT PDO Receive5/1 -> ModeofOperationDisplay/1
  DesireTorque/1 -> EtherCAT PDO Transmit/1
  EtherCAT PDO Receive1/1 -> ActuralPosition/1
  EtherCAT PDO Receive2/1 -> ActuralVelocity/1

== system Robot/Subsystem/Robot/Motor3 ==
  DesireTorque : Inport
  EtherCAT PDO Receive1 : slrealtimeethercatlib/EtherCAT PDO Receive  Priority=2  sig_name=Drive 3 (Elmo Drive ).Inputs.Position actual value  sig_offset=24784  sig_type=int32  type_size=32  sig_dim=1  device_id=0  sample_time=0.001000
  EtherCAT PDO Receive2 : slrealtimeethercatlib/EtherCAT PDO Receive  Priority=2  sig_name=Drive 3 (Elmo Drive ).Inputs_1.Velocity actual value  sig_offset=24864  sig_type=int32  type_size=32  sig_dim=1  device_id=0  sample_time=0.001000
  EtherCAT PDO Receive3 : slrealtimeethercatlib/EtherCAT PDO Receive  Priority=2  sig_name=Drive 3 (Elmo Drive ).Inputs.Torque actual value  sig_offset=24816  sig_type=int16  type_size=16  sig_dim=1  device_id=0  sample_time=0.001000
  EtherCAT PDO Receive4 : slrealtimeethercatlib/EtherCAT PDO Receive  Priority=2  sig_name=Drive 3 (Elmo Drive ).Inputs_2.DC link circuit voltage  sig_offset=24896  sig_type=uint32  type_size=32  sig_dim=1  device_id=0  sample_time=0.001000
  EtherCAT PDO Receive5 : slrealtimeethercatlib/EtherCAT PDO Receive  Priority=2  sig_name=Drive 3 (Elmo Drive ).Inputs.Mode of operation display  sig_offset=24848  sig_type=int8  type_size=8  sig_dim=1  device_id=0  sample_time=0.001000
  EtherCAT PDO Transmit : slrealtimeethercatlib/EtherCAT PDO Transmit  Priority=5  sig_name=Drive 3 (Elmo Drive ).Outputs.Target Torque  sig_offset=24784  sig_type=int16  type_size=16  sig_dim=1  device_id=0  sample_time=0.001000
  ActuralPosition : Outport
  ActuralVelocity : Outport  Port=2
  ActuralTorque : Outport  Port=3
  DCLinkCircuitVoltage : Outport  Port=4
  ModeofOperationDisplay : Outport  Port=5
  wires:
  EtherCAT PDO Receive4/1 -> DCLinkCircuitVoltage/1
  EtherCAT PDO Receive3/1 -> ActuralTorque/1
  EtherCAT PDO Receive5/1 -> ModeofOperationDisplay/1
  DesireTorque/1 -> EtherCAT PDO Transmit/1
  EtherCAT PDO Receive1/1 -> ActuralPosition/1
  EtherCAT PDO Receive2/1 -> ActuralVelocity/1

== system Robot/Subsystem/Robot/Motor4 ==
  DesireTorque : Inport
  EtherCAT PDO Receive1 : slrealtimeethercatlib/EtherCAT PDO Receive  Priority=2  sig_name=Drive 4 (Elmo Drive ).Inputs.Position actual value  sig_offset=39088  sig_type=int32  type_size=32  sig_dim=1  device_id=0  sample_time=0.001000
  EtherCAT PDO Receive2 : slrealtimeethercatlib/EtherCAT PDO Receive  Priority=2  sig_name=Drive 4 (Elmo Drive ).Inputs_1.Velocity actual value  sig_offset=39168  sig_type=int32  type_size=32  sig_dim=1  device_id=0  sample_time=0.001000
  EtherCAT PDO Receive3 : slrealtimeethercatlib/EtherCAT PDO Receive  Priority=2  sig_name=Drive 4 (Elmo Drive ).Inputs.Torque actual value  sig_offset=39120  sig_type=int16  type_size=16  sig_dim=1  device_id=0  sample_time=0.001000
  EtherCAT PDO Receive4 : slrealtimeethercatlib/EtherCAT PDO Receive  Priority=2  sig_name=Drive 4 (Elmo Drive ).Inputs_2.DC link circuit voltage  sig_offset=39200  sig_type=uint32  type_size=32  sig_dim=1  device_id=0  sample_time=0.001000
  EtherCAT PDO Receive5 : slrealtimeethercatlib/EtherCAT PDO Receive  Priority=2  sig_name=Drive 4 (Elmo Drive ).Inputs.Mode of operation display  sig_offset=39152  sig_type=int8  type_size=8  sig_dim=1  device_id=0  sample_time=0.001000
  EtherCAT PDO Transmit : slrealtimeethercatlib/EtherCAT PDO Transmit  Priority=5  sig_name=Drive 4 (Elmo Drive ).Outputs.Target Torque  sig_offset=39088  sig_type=int16  type_size=16  sig_dim=1  device_id=0  sample_time=0.001000
  ActuralPosition : Outport
  ActuralVelocity : Outport  Port=2
  ActuralTorque : Outport  Port=3
  DCLinkCircuitVoltage : Outport  Port=4
  ModeofOperationDisplay : Outport  Port=5
  wires:
  EtherCAT PDO Receive4/1 -> DCLinkCircuitVoltage/1
  EtherCAT PDO Receive3/1 -> ActuralTorque/1
  EtherCAT PDO Receive5/1 -> ModeofOperationDisplay/1
  DesireTorque/1 -> EtherCAT PDO Transmit/1
  EtherCAT PDO Receive1/1 -> ActuralPosition/1
  EtherCAT PDO Receive2/1 -> ActuralVelocity/1

== system Robot/Subsystem/Robot/STM32Device1 ==
  EtherCAT PDO Receive1 : slrealtimeethercatlib/EtherCAT PDO Receive  Priority=2  sig_name=Box 5 (PIC32 EtherCAT Slave01).INPUTS process data mapping.FORCE1  sig_offset=37072  sig_type=single  type_size=32  sig_dim=1  device_id=0  sample_time=0.001000
  EtherCAT PDO Receive2 : slrealtimeethercatlib/EtherCAT PDO Receive  Priority=2  sig_name=Box 5 (PIC32 EtherCAT Slave01).INPUTS process data mapping.FORCE2  sig_offset=37104  sig_type=single  type_size=32  sig_dim=1  device_id=0  sample_time=0.001000
  EtherCAT PDO Receive3 : slrealtimeethercatlib/EtherCAT PDO Receive  Priority=2  sig_name=Box 5 (PIC32 EtherCAT Slave01).INPUTS process data mapping.IMU1_X  sig_offset=37328  sig_type=single  type_size=32  sig_dim=1  device_id=0  sample_time=0.001000
  EtherCAT PDO Receive4 : slrealtimeethercatlib/EtherCAT PDO Receive  Priority=2  sig_name=Box 5 (PIC32 EtherCAT Slave01).INPUTS process data mapping.IMU1_Y  sig_offset=37360  sig_type=single  type_size=32  sig_dim=1  device_id=0  sample_time=0.001000
  EtherCAT PDO Receive5 : slrealtimeethercatlib/EtherCAT PDO Receive  Priority=2  sig_name=Box 5 (PIC32 EtherCAT Slave01).INPUTS process data mapping.IMU1_Z  sig_offset=37392  sig_type=single  type_size=32  sig_dim=1  device_id=0  sample_time=0.001000
  EtherCAT PDO Receive6 : slrealtimeethercatlib/EtherCAT PDO Receive  Priority=2  sig_name=Box 5 (PIC32 EtherCAT Slave01).INPUTS process data mapping.IMU2_X  sig_offset=37424  sig_type=single  type_size=32  sig_dim=1  device_id=0  sample_time=0.001000
  AD_Ch1 : Outport
  AD_Ch2 : Outport  Port=2
  Quaternions_q0 : Outport  Port=3
  Quaternions_q1 : Outport  Port=4
  Quaternions_q2 : Outport  Port=5
  Quaternions_q3 : Outport  Port=6
  wires:
  EtherCAT PDO Receive1/1 -> AD_Ch1/1
  EtherCAT PDO Receive4/1 -> Quaternions_q1/1
  EtherCAT PDO Receive5/1 -> Quaternions_q2/1
  EtherCAT PDO Receive3/1 -> Quaternions_q0/1
  EtherCAT PDO Receive6/1 -> Quaternions_q3/1
  EtherCAT PDO Receive2/1 -> AD_Ch2/1
